simulink model "BasicPolLPVmodel_Sat_sim"  (R2016a)
settings: Solver=ode45  StartTime=0.0  StopTime=5  MaxStep=0.01  RelTol=1e-3
libraries: lpvlibrary x6
settings Model: Creator=Fernando  LastModifiedBy=ferna

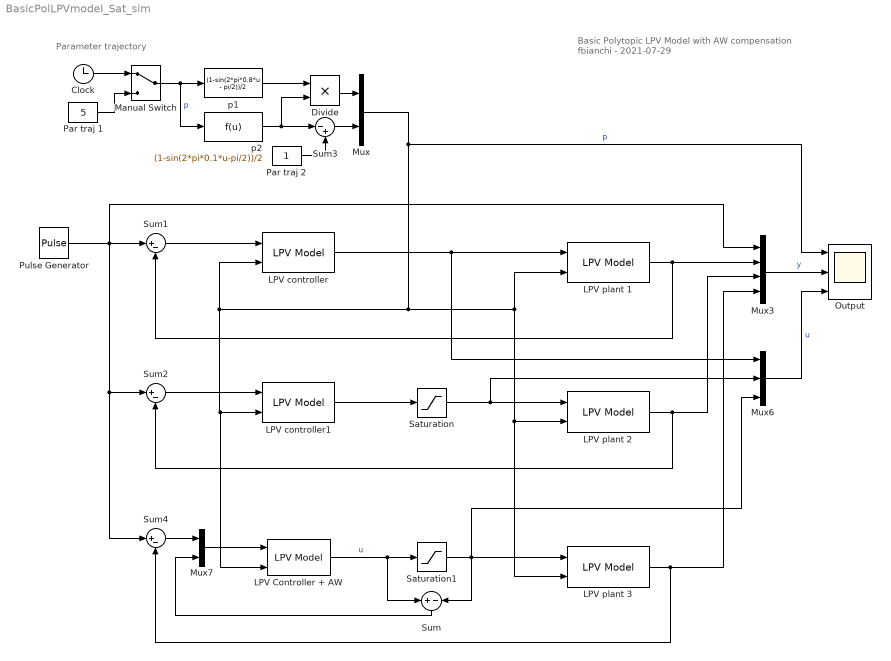
== system BasicPolLPVmodel_Sat_sim ==
  note: Basic Polytopic LPV Model with AW
      | compensation
      |
      | fbianchi - 2021-07-29
  note: Parameter trajectory
  Clock : Clock
  Divide : Product  Inputs=**
  LPV Controller + AW : lpvlibrary/LPV Model  pdSys=pdKaw  x0=0
  LPV controller : lpvlibrary/LPV Model  pdSys=pdK  x0=0
  LPV controller1 : lpvlibrary/LPV Model  pdSys=pdK  x0=0
  LPV plant 1 : lpvlibrary/LPV Model  pdSys=pdG  x0=0
  LPV plant 2 : lpvlibrary/LPV Model  pdSys=pdG  x0=0
  LPV plant 3 : lpvlibrary/LPV Model  pdSys=pdG  x0=0
  Manual Switch : ManualSwitch
  Mux : Mux  Inputs=2
  Mux3 : Mux
  Mux6 : Mux  Inputs=3
  Mux7 : Mux  Inputs=2
  Output : Scope  NumInputPorts=3
  Par traj 1 : Constant  Value=5
  Par traj 2 : Constant
  Pulse Generator : DiscretePulseGenerator  PulseType=Time based  Period=10  PulseWidth=25  PhaseDelay=0.5
  Saturation : Saturate  UpperLimit=0.2  LowerLimit=-0.2
  Saturation1 : Saturate  UpperLimit=0.2  LowerLimit=-0.2
  Sum : Sum  Inputs=+-
  Sum1 : Sum  Inputs=|+-
  Sum2 : Sum  Inputs=|+-
  Sum3 : Sum  Inputs=|-+
  Sum4 : Sum  Inputs=|+-
  p1 : Fcn  Expr=(1-sin(2*pi*0.8*u - pi/2))/2
  p2 : Fcn  Expr=(1-sin(2*pi*0.1*u-pi/2))/2
  wires:
  LPV controller/1 -> LPV plant 1/1, Mux6/1
  LPV plant 1/1 -> Sum1/2, Mux3/2
  Pulse Generator/1 -> Sum1/1, Sum2/1, Sum4/1, Mux3/1
  Sum2/1 -> LPV controller1/1
  LPV controller1/1 -> Saturation/1
  Saturation/1 -> LPV plant 2/1, Mux6/2
  Mux3/1 -> Output/2  "y"
  Mux6/1 -> Output/3  "u"
  LPV Controller + AW/1 -> Saturation1/1, Sum/1  "u"
  Saturation1/1 -> LPV plant 3/1, Sum/2, Mux6/3
  LPV plant 3/1 -> Sum4/2, Mux3/4
  Mux7/1 -> LPV Controller + AW/1
  Sum1/1 -> LPV controller/1
  LPV plant 2/1 -> Mux3/3, Sum2/2
  Manual Switch/1 -> p2/1, p1/1  "p"
  Clock/1 -> Manual Switch/1
  Par traj 1/1 -> Manual Switch/2
  p2/1 -> Sum3/1, Divide/2
  p1/1 -> Divide/1
  Par traj 2/1 -> Sum3/2
  Divide/1 -> Mux/1
  Sum3/1 -> Mux/2
  Mux/1 -> LPV Controller + AW/2, LPV controller1/2, LPV controller/2, LPV plant 1/2, LPV plant 2/2, LPV plant 3/2, Output/1  "p"
  Sum4/1 -> Mux7/1
  Sum/1 -> Mux7/2
